simulink model "fahrbahn1"  (Simulink 3.00)
settings: Solver=ode45  StartTime=0.0  StopTime=10.0  RelTol=1e-3
settings Model: LastModifiedBy=student

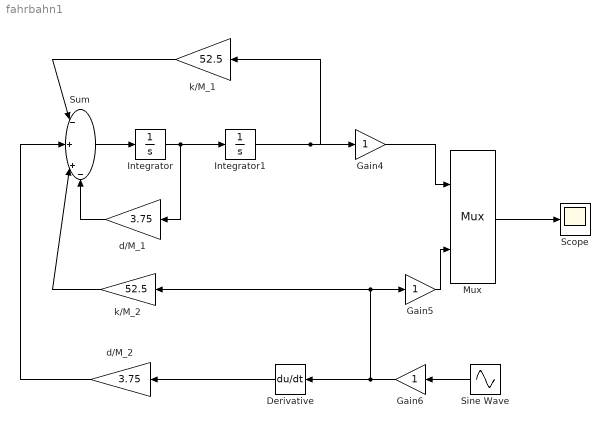
== system fahrbahn1 ==
  Derivative : Derivative  Orientation=left
  Gain4 : Gain  Gain=1  SaturateOnIntegerOverflow=on
  Gain5 : Gain  Gain=1  SaturateOnIntegerOverflow=on
  Gain6 : Gain  Orientation=left  Gain=1  SaturateOnIntegerOverflow=on
  Integrator : Integrator  ExternalReset=none  InitialConditionSource=internal  InitialCondition=0  LimitOutput=off  UpperSaturationLimit=inf  LowerSaturationLimit=-inf  ShowSaturationPort=off  ShowStatePort=off  AbsoluteTolerance=auto
  Integrator1 : Integrator  ExternalReset=none  InitialConditionSource=internal  InitialCondition=0  LimitOutput=off  UpperSaturationLimit=inf  LowerSaturationLimit=-inf  ShowSaturationPort=off  ShowStatePort=off  AbsoluteTolerance=auto
  Mux : Mux  Inputs=2
      settings: DisplayOption=signals
  Scope : Scope
      settings: TimeRange=1  YMin=0  YMax=1  SaveToWorkspace=off  SaveName=ScopeData
  Sine Wave : Sin  Orientation=left  Amplitude=0.1  Frequency=6.28  Phase=0  SampleTime=0
  Sum : Sum  Inputs=|-++-  SaturateOnIntegerOverflow=on
  d/M_1 : Gain  Orientation=left  Gain=3.75  SaturateOnIntegerOverflow=on
  d/M_2 : Gain  Orientation=left  Gain=3.75  SaturateOnIntegerOverflow=on
  k/M_1 : Gain  Orientation=left  Gain=52.5  SaturateOnIntegerOverflow=on
  "k/M_2 " : Gain  Orientation=left  Gain=52.5  SaturateOnIntegerOverflow=on
  wires:
  Derivative/1 -> d/M_2/1
  Integrator/1 -> Integrator1/1, d/M_1/1
  d/M_1/1 -> Sum/4
  "k/M_2 "/1 -> Sum/3
  d/M_2/1 -> Sum/2
  k/M_1/1 -> Sum/1
  Sum/1 -> Integrator/1
  Integrator1/1 -> k/M_1/1, Gain4/1
  Gain4/1 -> Mux/1
  Gain5/1 -> Mux/2
  Mux/1 -> Scope/1
  Sine Wave/1 -> Gain6/1
  Gain6/1 -> Derivative/1, Gain5/1, "k/M_2 "/1
